simulink model "B_2025"  (R2024b)
settings: Solver=ode23t  StartTime=0.0  StopTime=5  RelTol=1e-3
InitFcn:
  | Ts=1e-5;
  | 
  | % Rectifier AC side :
  | VLL_nom_R = 500e3; % V
  | Fnom_R = 50;           % Hz
  | 
  | % Inverter AC side :
  | VLL_nom_I = 345e3; % V
  | Fnom_I = 50;           % Hz
  | 
  | % DC :
  | Vdc_nom = 500e3;   % V
  | Idc_nom  = 2000;     % A
  | Ts_c=50e-6;
  | Freq_filter=10000;
  | Zeta_filter=1;
  | kSOGI=1.414;
libraries: spsSeriesRLCBranchLib x6, spsDiodeLib x4, spsMosfetLib x4, spsCurrentMeasurementLib x3, spsSecondOrderFilterLib x3, spsACVoltageSourceLib x1, spsDCVoltageSourceLib x1, spsPLLLib x1, spsRMSLib x1, simulink x1, spsVoltageMeasurementLib x1, sps_lib x1
settings Model: Creator=17332  LastModifiedBy=26279
settings DataIOCC: ReturnWorkspaceOutputs=off

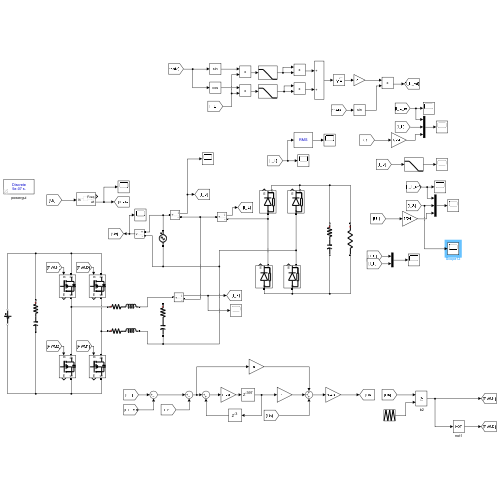
[thumbnail: Simulink's stored preview of the top-level diagram]
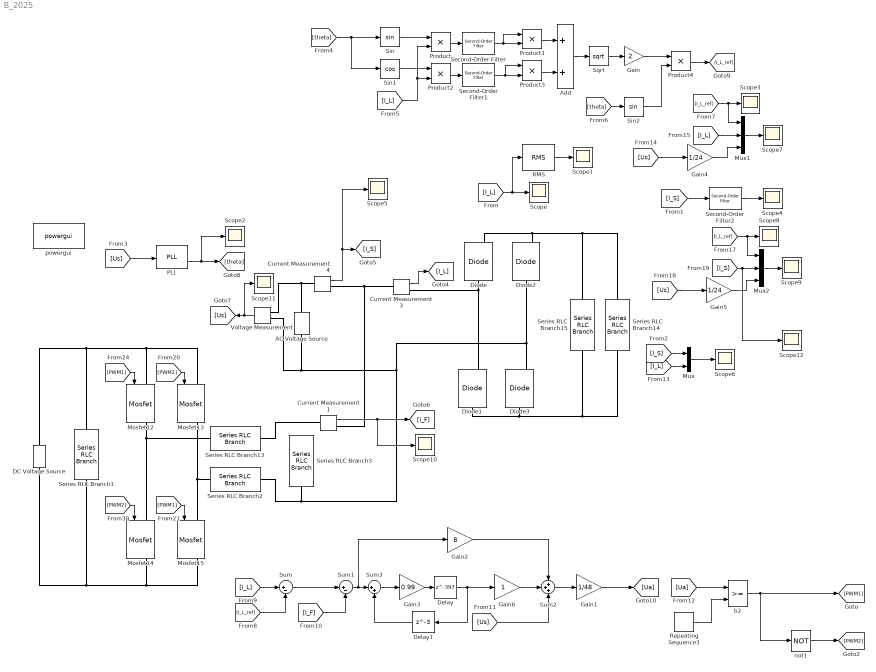
== system B_2025 ==
  " b2" : RelationalOperator  OutDataTypeStr=boolean  InputSameDT=off
  AC Voltage Source : spsACVoltageSourceLib/AC Voltage Source  Amplitude=24  Phase=0  Frequency=50  SampleTime=0  Measurements=None  BusType=swing  Pref=10e3  Qref=0  Qmin=-inf  Qmax=+inf
  Add : Sum
  Current Measurement1 : spsCurrentMeasurementLib/Current Measurement  PhasorSimulation=off  OutputType=Complex  PSBequivalent=0
  Current Measurement3 : spsCurrentMeasurementLib/Current Measurement  PhasorSimulation=off  OutputType=Complex  PSBequivalent=0
  Current Measurement4 : spsCurrentMeasurementLib/Current Measurement  PhasorSimulation=off  OutputType=Complex  PSBequivalent=0
  DC Voltage Source : spsDCVoltageSourceLib/DC Voltage Source  Amplitude=48  Measurements=None
  Delay : Delay  DelayLength=397
  Delay1 : Delay  DelayLength=3
  Diode{,1..3} (4 alike) : spsDiodeLib/Diode  Ron=0.001  Lon=0  Vf=0.8  IC=0  UseSnubber=0  Rs=500  Cs=250e-9  Measurements=on
  Gain : Gain  Gain=2
  Gain1 : Gain  Gain=1/48
  Gain2 : Gain  Gain=8
  Gain3 : Gain  Gain=0.99
  Gain4 : Gain  Gain=1/24
  Gain5 : Gain  Gain=1/24
  Gain6 : Gain
  Mosfet{12..15} (4 alike) : spsMosfetLib/Mosfet  Ron=0.01  Lon=0  Rd=0.01  Vfd=0  IC=0  Rs=1e5  Cs=inf  Measurements=on
  Mux : Mux  Inputs=2
  Mux1 : Mux  Inputs=3
  Mux2 : Mux  Inputs=3
  PLL : spsPLLLib/PLL  Fmin=45  Par_Init=[0, 50]  ParK=[180, 3200, 1]  TcD=1e-4  MaxRateChangeFreq=12  FilterCutOffFreq=25  Ts=0  AGC=on
      settings: LibrarySourceBlock=sps_lib/Control/PLL
  Product{,1..4} (5 alike) : Product
  RMS : spsRMSLib/RMS  TrueRMS=on  Freq=50  RMSInit=2  Ts=0
  Repeating Sequence3 : simulink/Sources/Repeating Sequence  rep_seq_t=[0 1/2 1]/40000  rep_seq_y=[-0.5 0.5 -0.5]
  Scope{,1..12} (13 alike) : Scope
  Second-Order Filter : spsSecondOrderFilterLib/Second-Order Filter  FilterType=Lowpass  Fo=5  Zeta=0.707  Ts=0  Initialize=off  Vac_Init="[0,  0,  60]"  Vdc_Init=0.94  PlotResponse=off  FreqRange=[0, 500, 1]
      settings: LibrarySourceBlock=|
      | sps_lib/Control/Filters/Second-Order
      | Filter
  Second-Order Filter1 : spsSecondOrderFilterLib/Second-Order Filter  FilterType=Lowpass  Fo=5  Zeta=0.707  Ts=0  Initialize=off  Vac_Init="[0,  0,  60]"  Vdc_Init=0.41  PlotResponse=off  FreqRange=[0, 500, 1]
      settings: LibrarySourceBlock=|
      | sps_lib/Control/Filters/Second-Order
      | Filter
  Second-Order Filter2 : spsSecondOrderFilterLib/Second-Order Filter  FilterType=Lowpass  Fo=3000  Zeta=0.707  Ts=0  Initialize=off  Vac_Init="[0,  0,  60]"  Vdc_Init=0.94  PlotResponse=off  FreqRange=[0, 500, 1]
      settings: LibrarySourceBlock=|
      | sps_lib/Control/Filters/Second-Order
      | Filter
  Series RLC Branch1 : spsSeriesRLCBranchLib/Series RLC Branch  LConnTagsString=__new0  RConnTagsString=__new0  BranchType=RC  Resistance=0.2  Inductance=220e-6  SetiL0=off  InitialCurrent=0  Capacitance=1000e-6  Setx0=on  InitialVoltage=48  Measurements=None
  Series RLC Branch13 : spsSeriesRLCBranchLib/Series RLC Branch  LConnTagsString=__new0  RConnTagsString=__new0  BranchType=RL  Resistance=0.2  Inductance=220e-6  SetiL0=off  InitialCurrent=0  Capacitance=1e-6  Setx0=off  InitialVoltage=0  Measurements=None
  Series RLC Branch14 : spsSeriesRLCBranchLib/Series RLC Branch  LConnTagsString=__new0  RConnTagsString=__new0  BranchType=R  Resistance=18  Inductance=220e-6  SetiL0=off  InitialCurrent=0  Capacitance=1e-6  Setx0=off  InitialVoltage=0  Measurements=None
  Series RLC Branch15 : spsSeriesRLCBranchLib/Series RLC Branch  LConnTagsString=__new0  RConnTagsString=__new0  BranchType=RC  Resistance=0.2  Inductance=220e-6  SetiL0=off  InitialCurrent=0  Capacitance=1000e-6  Setx0=off  InitialVoltage=0  Measurements=None
  Series RLC Branch2 : spsSeriesRLCBranchLib/Series RLC Branch  LConnTagsString=__new0  RConnTagsString=__new0  BranchType=RL  Resistance=0.2  Inductance=220e-6  SetiL0=off  InitialCurrent=0  Capacitance=1e-6  Setx0=off  InitialVoltage=0  Measurements=None
  Series RLC Branch3 : spsSeriesRLCBranchLib/Series RLC Branch  LConnTagsString=__new0  RConnTagsString=__new0  BranchType=RC  Resistance=100  Inductance=220e-6  SetiL0=off  InitialCurrent=0  Capacitance=40e-6  Setx0=off  InitialVoltage=48  Measurements=None
  Sin : Trigonometry
  Sin1 : Trigonometry  Operator=cos
  Sin2 : Trigonometry
  Sqrt : Sqrt
  Sum : Sum  Inputs=|+-
  Sum1 : Sum  Inputs=|+-
  Sum2 : Sum  Inputs=+++
  Sum3 : Sum  Inputs=|++
  Voltage Measurement : spsVoltageMeasurementLib/Voltage Measurement  PhasorSimulation=off  OutputType=Complex  PSBequivalent=0
  not1 : Logic  Operator=NOT  AllPortsSameDT=off  OutDataTypeStr=boolean
  powergui : sps_lib/powergui  Priority=1  SimulationMode=Discrete  SampleTime=5e-7  frequency=60  Iterations=50  frequencyindice=50  Pbase=100e6  ErrMax=1e-4  UnitsV=kV  UnitsW=MW  buscounter=0  FunctionMessages=off  echomessages=off  EnableUseOfTLC=off  CurrentSourceSwitches=off  DisableSnubberDevices=off  DisableRonSwitches=off  DisableVfSwitches=off  DisplayEquations=off  AutomaticDiscreteSolvers=off  SolverType=Tustin/Backward Euler (TBE)  Interpol=off  ExternalGateDelay=off  methode=off  Ts=100  x0status=blocks  SPID=on  SwTol=0  HookPort=off  NonlinearTolerance=1e-4  nMaxIteration=100  ContinueOnMaxIteration=off  RestoreLinks=warning  ResistiveCurrentMeasurement=off  Frange=[0:2:500]  Ylog=off  Xlog=on  ShowGrid=off  save=off  variable=ZData  structure=0  ZoomFFT=off  StartTime=0.0  cycles=1  DisplayStyle=1  fundamental=60  FreqAxis=off  MaxFrequency=1000  frequencyindicesteady=1  RmsSteady=1  display=off
  wires:
  [PWM2] -> Mosfet14/1
  [PWM1] -> Mosfet12/1
  [PWM1] -> Mosfet15/1
  [PWM2] -> Mosfet13/1
  Current Measurement3/1 -> [I_L]
  [I_L] -> RMS/1, Scope/1
  RMS/1 -> Scope1/1
  Current Measurement4/1 -> [I_S], Scope5/1
  Current Measurement1/1 -> Scope10/1, [I_F]
  Voltage Measurement/1 -> Scope11/1, [Us]
  [Us] -> PLL/1
  PLL/2 -> Scope2/1, [theta]
  [theta] -> Sin1/1, Sin/1
  Sin/1 -> Product/1
  Sin1/1 -> Product2/1
  [I_L] -> Product/2, Product2/2
  Product/1 -> Second-Order Filter/1
  Product2/1 -> Second-Order Filter1/1
  Second-Order Filter/1 -> Product1/1, Product1/2
  Second-Order Filter1/1 -> Product3/1, Product3/2
  Product3/1 -> Add/2
  Product1/1 -> Add/1
  Add/1 -> Sqrt/1
  Sqrt/1 -> Gain/1
  [theta] -> Sin2/1
  Gain/1 -> Product4/1
  Sin2/1 -> Product4/2
  Product4/1 -> [I_L_ref]
  [I_L_ref] -> Mux1/1, Scope3/1
  [I_L] -> Sum/1
  [I_L_ref] -> Sum/2
  Sum/1 -> Sum1/1
  [I_F] -> Sum1/2
  Sum2/1 -> Gain1/1
  [Us] -> Sum2/3
  Gain2/1 -> Sum2/1
  Sum1/1 -> Sum3/1, Gain2/1
  Gain1/1 -> [Ua]
  [Ua] -> " b2"/1
  Repeating Sequence3/1 -> " b2"/2
  " b2"/1 -> not1/1, [PWM1]
  not1/1 -> [PWM2]
  Gain3/1 -> Delay/1
  Delay/1 -> Gain6/1, Delay1/1
  Delay1/1 -> Sum3/2
  Sum3/1 -> Gain3/1
  [I_S] -> Second-Order Filter2/1
  Second-Order Filter2/1 -> Scope4/1
  Mux/1 -> Scope6/1
  [I_S] -> Mux/1
  [I_L] -> Mux/2
  [I_L] -> Mux1/2
  Mux1/1 -> Scope7/1
  [Us] -> Gain4/1
  Gain4/1 -> Mux1/3
  [I_S] -> Scope12/1, Mux2/2
  [I_L_ref] -> Mux2/1, Scope8/1
  Gain5/1 -> Mux2/3
  [Us] -> Gain5/1
  Mux2/1 -> Scope9/1
  Gain6/1 -> Sum2/2
  connections:
  Mosfet14/LConn1 -- Series RLC Branch13/LConn1 -- Mosfet12/RConn1
  Mosfet15/LConn1 -- Series RLC Branch2/LConn1 -- Mosfet13/RConn1
  Current Measurement4/LConn1 -- AC Voltage Source/RConn1 -- Voltage Measurement/LConn1
  Current Measurement4/RConn1 -- Current Measurement1/RConn1 -- Current Measurement3/LConn1
  Diode1/RConn1 -- Current Measurement3/RConn1 -- Diode/LConn1
  Diode3/RConn1 -- Voltage Measurement/LConn2 -- AC Voltage Source/LConn1 -- Series RLC Branch3/RConn1 -- Series RLC Branch2/RConn1 -- Diode2/LConn1
  Diode/RConn1 -- Series RLC Branch14/LConn1 -- Series RLC Branch15/LConn1 -- Diode2/RConn1
  Diode1/LConn1 -- Series RLC Branch14/RConn1 -- Series RLC Branch15/RConn1 -- Diode3/LConn1
  DC Voltage Source/RConn1 -- Series RLC Branch1/LConn1 -- Mosfet12/LConn1 -- Mosfet13/LConn1
  DC Voltage Source/LConn1 -- Series RLC Branch1/RConn1 -- Mosfet15/RConn1 -- Mosfet14/RConn1
  Current Measurement1/LConn1 -- Series RLC Branch13/RConn1
